simulink model "result1"  (R2020a)
settings: Solver=VariableStepAuto  StartTime=0.0  StopTime=10.0  RelTol=1e-3
settings Model: Creator=ASUS  LastModifiedBy=ASUS

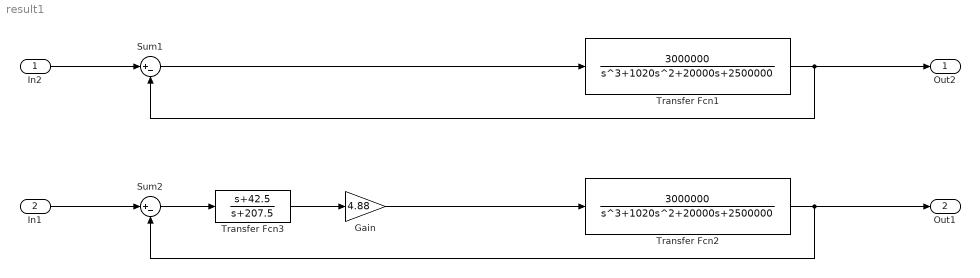
== system result1 ==
  In2 : Inport
  In1 : Inport  Port=2
  Gain : Gain  Gain=4.88
  Sum1 : Sum  Inputs=|+-
  Sum2 : Sum  Inputs=|+-
  Transfer Fcn1 : TransferFcn  Numerator=[3000000]  Denominator=[1 1020 20000 2500000]
  Transfer Fcn2 : TransferFcn  Numerator=[3000000]  Denominator=[1 1020 20000 2500000]
  Transfer Fcn3 : TransferFcn  Numerator=[1 42.5]  Denominator=[1 207.5]
  Out2 : Outport
  Out1 : Outport  Port=2
  wires:
  Transfer Fcn1/1 -> Out2/1, Sum1/2
  Sum1/1 -> Transfer Fcn1/1
  In2/1 -> Sum1/1
  Sum2/1 -> Transfer Fcn3/1
  In1/1 -> Sum2/1
  Transfer Fcn2/1 -> Out1/1, Sum2/2
  Gain/1 -> Transfer Fcn2/1
  Transfer Fcn3/1 -> Gain/1
